simulink model "model1"  (R2022b)
settings: Solver=FixedStepAuto  StartTime=0.0  StopTime=10.0  FixedStep=0.01  RelTol=1e-3
undefined symbols (not defined in the file): NULL
libraries: instrumentseriallib x2
settings Model: Creator=Aleksandr  LastModifiedBy=Aleksandr
settings DebuggingCC: UnconnectedInputMsg=warning  UnconnectedOutputMsg=warning  UnconnectedLineMsg=warning
settings ModelReferenceCC: EnableRefExpFcnMdlSchedulingChecks=on
settings RTWCC: DLArmComputeVersion=19.05

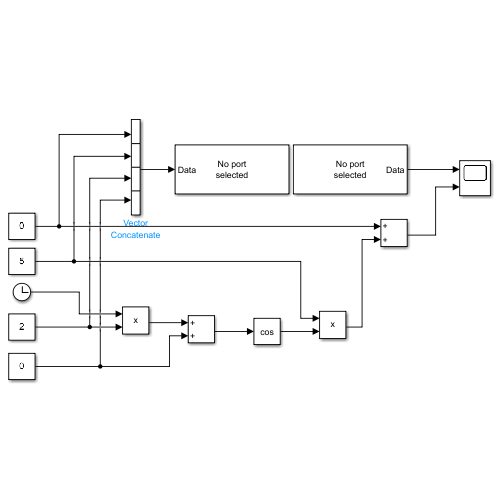
[thumbnail: Simulink's stored preview of the top-level diagram]
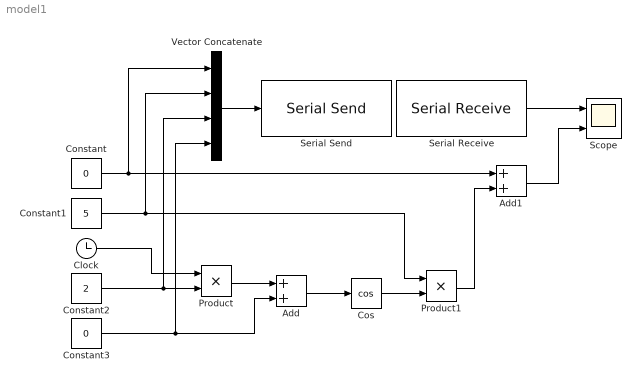
== system model1 ==
  Add : Sum
  Add1 : Sum
  Clock : Clock
  Constant : Constant  Value=0
  Constant1 : Constant  Value=5
  Constant2 : Constant  Value=2
  Constant3 : Constant  Value=0
  Cos : Trigonometry  Operator=cos
  Product : Product
  Product1 : Product
  Scope : Scope  NumInputPorts=2
  Serial Receive : instrumentseriallib/Serial Receive  Priority=1  PortSel=<Select a port...>  Port=<Select a port...>  ComPort=<Select a port...>  DataType=single  SaveDataType=uint8  ToggleHeader=off  Header=['b']  ToggleTerminator=off  Terminator=NULL ('\0')  CustomTerminator=[]  InputFormat=Column major  ToggleDataSize=on  DataSize=[1 1]  EnableBlockingMode=on  ActionDataUnavailable=Output last received value  ActionWhenDataUnavailable=Output last received value  CustomValue=0  SampleTime=0.01  SimulateUsing=Interpreted execution  BlockInModel=on  aMode=1
  Serial Send : instrumentseriallib/Serial Send  Priority=1  PortSel=<Select a port...>  Port=<Select a port...>  ComPort=<Select a port...>  Header=[]  Terminator=<none>  CustomTerminator=[]  EnableBlockingMode=on  SimulateUsing=Interpreted execution  BlockInModel=on  aMode=1
  Vector Concatenate : Concatenate  NumInputs=4
  wires:
  Constant2/1 -> Product/2, Vector Concatenate/3
  Clock/1 -> Product/1
  Product/1 -> Add/1
  Constant3/1 -> Add/2, Vector Concatenate/4
  Add/1 -> Cos/1
  Cos/1 -> Product1/2
  Constant1/1 -> Product1/1, Vector Concatenate/2
  Constant/1 -> Add1/1, Vector Concatenate/1
  Product1/1 -> Add1/2
  Serial Receive/1 -> Scope/1
  Add1/1 -> Scope/2
  Vector Concatenate/1 -> Serial Send/1
